simulink model "Plotter"  (R2018a)
settings: Solver=FixedStepAuto  StartTime=0.0  StopTime=10.0  FixedStep=10e-4  RelTol=1e-3
values from neighbouring files (symbols this model uses):
  rEmax = 0.067    [SmaParameters.m]
undefined symbols (not defined in the file or in its folder): austRecoveryArray, lkpAustStressRange, lkpAustTempRange, lkpMartStrainRange, lkpMartTempRange, martDetwiningArray
settings Model: Creator=Michau  LastModifiedBy=Michau
settings SolverCC: AlgebraicLoopSolver=LineSearch

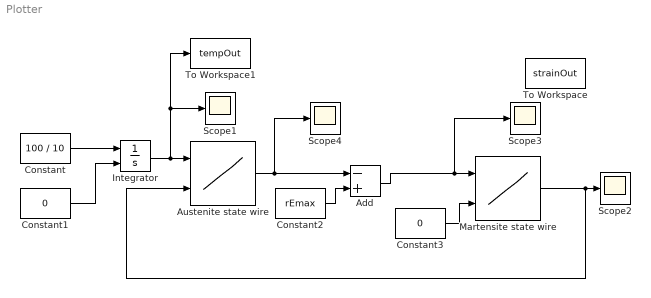
== system Plotter ==
  Add : Sum  Inputs=-+
  Austenite state wire : Lookup_n-D  BreakpointsForDimension1=lkpAustTempRange  BreakpointsForDimension2=lkpAustStressRange  Table=austRecoveryArray  ExtrapMethod=Clip  UseLastTableValue=on  InternalRulePriority=Speed  RndMeth=Simplest  InputSameDT=on
  Constant : Constant  Value=100 / 10
  Constant1 : Constant  Value=0
  Constant2 : Constant  Value=rEmax
  Constant3 : Constant  Value=0
  Integrator : Integrator  InitialConditionSource=external
  Martensite state wire : Lookup_n-D  BreakpointsForDimension1=lkpMartStrainRange  BreakpointsForDimension2=lkpMartTempRange  Table=martDetwiningArray  InternalRulePriority=Speed  RndMeth=Simplest  InputSameDT=on
  Scope{1..4} (4 alike) : Scope
  To Workspace : ToWorkspace  VariableName=strainOut  SampleTime=-1
  To Workspace1 : ToWorkspace  VariableName=tempOut  SampleTime=-1
  wires:
  Constant/1 -> Integrator/1
  Constant1/1 -> Integrator/2
  Integrator/1 -> Scope1/1, To Workspace1/1, Austenite state wire/1
  Constant3/1 -> Martensite state wire/2
  Martensite state wire/1 -> Austenite state wire/2, Scope2/1
  Add/1 -> Scope3/1, Martensite state wire/1
  Austenite state wire/1 -> Scope4/1, Add/1
  Constant2/1 -> Add/2
